simulink model "System_with_Robot"  (R2015b)
settings: Solver=FixedStepAuto  StartTime=0.0  StopTime=10.0  FixedStep=0.1  RelTol=1e-3
settings Model: Creator=Deepak  LastModifiedBy=Deepak

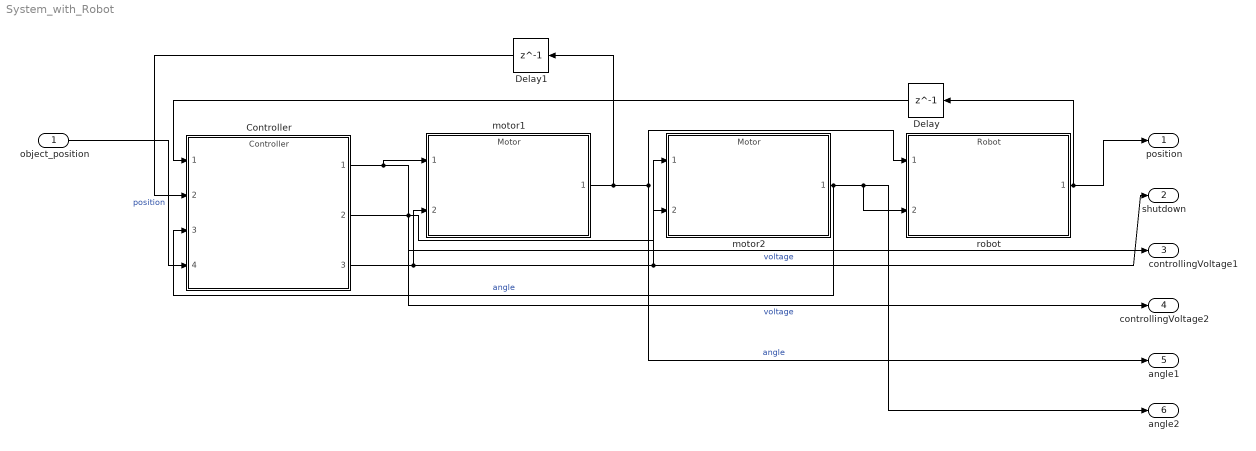
== system System_with_Robot ==
  object_position : Inport
      settings: AttributesFormatString=position
  Controller : ModelReference  ModelNameDialog=Controller  SimulationMode=Normal  ModelReferenceVersion=1.37  CopyOfModelName=Controller
  Delay : Delay  DelayLength=1  InitialCondition=[0,0]
  Delay1 : Delay  DelayLength=1  InitialCondition=0
  motor1 : ModelReference  ModelNameDialog=Motor  SimulationMode=Normal  ModelReferenceVersion=1.7  CopyOfModelName=Motor
  motor2 : ModelReference  ModelNameDialog=Motor  SimulationMode=Normal  ModelReferenceVersion=1.7  CopyOfModelName=Motor
  robot : ModelReference  ModelNameDialog=Robot  SimulationMode=Normal  ModelReferenceVersion=1.4  CopyOfModelName=Robot
  position : Outport
  shutdown : Outport  Port=2
  controllingVoltage1 : Outport  Port=3
      settings: AttributesFormatString=voltage
  controllingVoltage2 : Outport  Port=4
      settings: AttributesFormatString=voltage
  angle1 : Outport  Port=5
      settings: AttributesFormatString=angle
  angle2 : Outport  Port=6
      settings: AttributesFormatString=angle
  wires:
  Controller/1 -> motor1/1, controllingVoltage1/1  "voltage"
  Controller/2 -> motor2/1, controllingVoltage2/1  "voltage"
  Controller/3 -> motor2/2, shutdown/1, motor1/2
  motor1/1 -> Delay1/1, robot/1, angle1/1  "angle"
  motor2/1 -> robot/2, angle2/1, Controller/3  "angle"
  robot/1 -> Delay/1, position/1
  object_position/1 -> Controller/4  "position"
  Delay/1 -> Controller/1
  Delay1/1 -> Controller/2
